simulink model "Simulacion_a"  (R2021a)
settings: Solver=VariableStepAuto  StartTime=0.0  StopTime=50000.0  RelTol=1e-3
values from neighbouring files (symbols this model uses):
  Qi = 8/(1000*60)    (= 0.000133333333333)    [TP1.m]
  ue = double(ue)    [TP1.m]
  x1e = 0.45    [TP1.m]
  ye = 0.45    [TP1.m]
libraries: cstblocks x1
settings Model: Creator=amddy  LastModifiedBy=Usuario

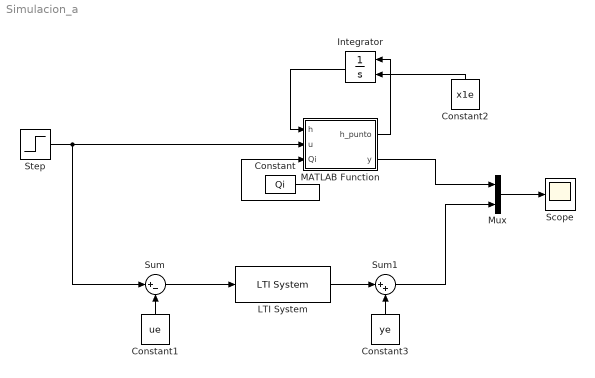
== system Simulacion_a ==
  Constant : Constant  Value=Qi
  Constant1 : Constant  Value=ue
  Constant2 : Constant  Value=x1e
  Constant3 : Constant  Value=ye
  Integrator : Integrator  InitialConditionSource=external
  LTI System : cstblocks/LTI System  sys=G  IC=[]
  MATLAB Function : MATLAB Function  TreatAsAtomicUnit=on
  Mux : Mux  Inputs=2
  Scope : Scope
  Step : Step  Time=20000  Before=ue  After=ue*1.1  SampleTime=0
  Sum : Sum  Inputs=|+-
  Sum1 : Sum  Inputs=|++
  wires:
  Integrator/1 -> MATLAB Function/1(h)
  Constant/1 -> MATLAB Function/3(Qi)
  MATLAB Function/1(h_punto) -> Integrator/1
  Step/1 -> Sum/1, MATLAB Function/2(u)
  Mux/1 -> Scope/1
  Constant2/1 -> Integrator/2
  Constant1/1 -> Sum/2
  Sum/1 -> LTI System/1
  LTI System/1 -> Sum1/1
  MATLAB Function/2(y) -> Mux/1
  Sum1/1 -> Mux/2
  Constant3/1 -> Sum1/2

== matlab function Simulacion_a/MATLAB Function ==
  data: h input; h_punto output; u input; Qi input; y output
function [h_punto,y] = fcn(h,u,Qi)

d_tuberia= 10.65e-3; % metros
lb = 10e-2;  % metros
la= 40e-2; % metros
S= pi*((d_tuberia/2)^2); % metros^2
L=0.9; % metros
g=9.81; % metros/seg^2

h_punto= (Qi - S*u*sqrt(2*g*h))/(lb + (la - lb)*h/L);
y=h;
end
